simulink model "passive_filters"  (R2016a)
settings: Solver=ode23t  StartTime=0.0  StopTime=0.1  RelTol=1e-3  AbsTol=1e-3
libraries: fl_lib x60, nesl_utility x39
settings Model: Creator=marin  LastModifiedBy=marin
settings DataIOCC: LimitDataPoints=on
settings DebuggingCC: AllowSymbolicDim=off
settings ConfigComp: CovModelRefEnable=Off  CovSFcnEnable=off
settings SimscapeCC: SimscapeLogType=all  SimscapeLogDataHistory=10000

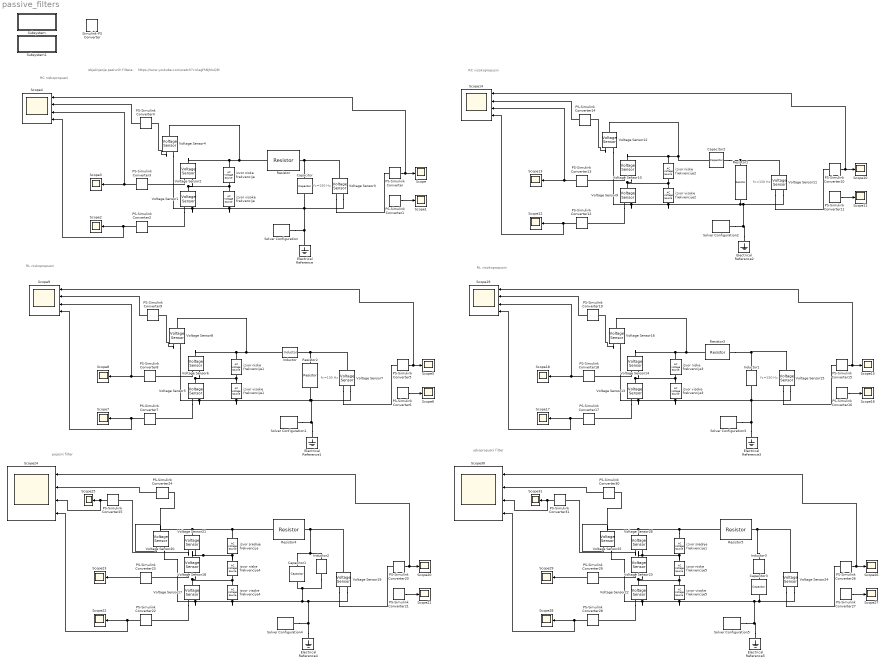
== system passive_filters ==
  note: uskopropusni filter
  note: pojasni filter
  note: RC visokopropusni
  note: RL niskopropusni
  note: RC niskopropusni
  note: objašnjenje pasivnih filtera:
  note: https://www.youtube.com/watch?v=lagfhNjMuQM
  note: fc=150 Hz
  note: fc=150 Hz
  note: fc=150 Hz
  note: RL visokopropusni
  note: fc=150 Hz
  Capacitor : fl_lib/Electrical/Electrical Elements/Capacitor  c=0.0011 F  r=1e-6 Ohm  g=0 1/Ohm  i_specify=off  i_priority=None  i=0 A  v_specify=off  v_priority=None  v=0 V  vc_specify=off  vc_priority=High  vc=0 V
  Capacitor1 : fl_lib/Electrical/Electrical Elements/Capacitor  c=0.0032 F  r=1e-6 Ohm  g=0 1/Ohm  i_specify=off  i_priority=None  i=0 A  v_specify=off  v_priority=None  v=0 V  vc_specify=off  vc_priority=High  vc=0 V
  Capacitor2 : fl_lib/Electrical/Electrical Elements/Capacitor  c=0.0011 F  r=1e-6 Ohm  g=0 1/Ohm  i_specify=off  i_priority=None  i=0 A  v_specify=off  v_priority=None  v=0 V  vc_specify=off  vc_priority=High  vc=0 V
  Capacitor3 : fl_lib/Electrical/Electrical Elements/Capacitor  c=0.0032 F  r=1e-6 Ohm  g=0 1/Ohm  i_specify=off  i_priority=None  i=0 A  v_specify=off  v_priority=None  v=0 V  vc_specify=off  vc_priority=High  vc=0 V
  Electrical Reference{,1..5} (6 alike) : fl_lib/Electrical/Electrical Elements/Electrical Reference
  Inductor : fl_lib/Electrical/Electrical Elements/Inductor  l=1e-6 H  r=0 Ohm  g=1e-9 1/Ohm  i_specify=off  i_priority=None  i=0 A  v_specify=off  v_priority=None  v=0 V  i_L_specify=off  i_L_priority=High  i_L=0 A
  Inductor1 : fl_lib/Electrical/Electrical Elements/Inductor  l=1e-6 H  r=0 Ohm  g=1e-9 1/Ohm  i_specify=off  i_priority=None  i=0 A  v_specify=off  v_priority=None  v=0 V  i_L_specify=off  i_L_priority=High  i_L=0 A
  Inductor2 : fl_lib/Electrical/Electrical Elements/Inductor  l=1.9894e-04 H  r=0 Ohm  g=1e-9 1/Ohm  i_specify=off  i_priority=None  i=0 A  v_specify=off  v_priority=None  v=0 V  i_L_specify=off  i_L_priority=High  i_L=0 A
  Inductor3 : fl_lib/Electrical/Electrical Elements/Inductor  l=1.9894e-04 H  r=0 Ohm  g=1e-9 1/Ohm  i_specify=off  i_priority=None  i=0 A  v_specify=off  v_priority=None  v=0 V  i_L_specify=off  i_L_priority=High  i_L=0 A
  PS-Simulink Converter{,1..31} (32 alike) : nesl_utility/PS-Simulink Converter  PhysicalDomain=network_engine_domain  SubClassName=ps_output  LeftPortType=input  RightPortType=output  PseudoPeriodic=off  Frequencies=[]  Unit=1  AffineConversion=off
  Resistor{,1,4..5} (4 alike) : fl_lib/Electrical/Electrical Elements/Resistor  R=1 Ohm  i_specify=off  i_priority=None  i=0 A  v_specify=off  v_priority=None  v=0 V
  Resistor2 : fl_lib/Electrical/Electrical Elements/Resistor  R=0.0011 Ohm  i_specify=off  i_priority=None  i=0 A  v_specify=off  v_priority=None  v=0 V
  Resistor3 : fl_lib/Electrical/Electrical Elements/Resistor  R=0.0011 Ohm  i_specify=off  i_priority=None  i=0 A  v_specify=off  v_priority=None  v=0 V
  Scope{,1..3,5..8,10..13,15..18,20..23,25..29,31} (26 alike) : Scope
  Scope{4,9,14,19,24,30} (6 alike) : Scope  NumInputPorts=4
  Simulink-PS Converter : nesl_utility/Simulink-PS Converter  PhysicalDomain=network_engine_domain  SubClassName=ps_input  LeftPortType=input  RightPortType=output  PseudoPeriodic=off  Frequencies=[]  NoiseDistribution=none  NoiseParameters=[]  Unit=1  AffineConversion=off  InputFiltering=off  SimscapeFilterOrder=1  InputFilterTimeConstant=0.001  UdotUserProvided=1
  Solver Configuration{,1..5} (6 alike) : nesl_utility/Solver Configuration  PhysicalDomain=network_engine_domain  SubClassName=solver  LeftPortType=input  RightPortType=generic  Accelerate=off  Tones=[]  Harmonics=[]  SimulateNoise=off  Profile=off  UseLocalSampling=off  EnableSwitchedLinearOptims=on  FrequencyDomain=off  UseCCode=off  RelTol=0.001  AbsTol=1e-06  MinStep=1e-09  ToWorkspace=off  RevertToSquareIcSolve=off  NumHomotopyIterations=100  PhasorMode=off  PhasorModeNumHarmonics=1  OverrideAbsTol=off  DoDC=off  ResidualTolerance=1e-09  UseLocalSolver=off  LocalSolverChoice=NE_BACKWARD_EULER_ADVANCER  LocalSolverSampleTime=0.001  DoFixedCost=off  MaxNonlinIter=3  MaxModeIter=2  LinearAlgebra=Sparse  DelaysMemoryBudget=1024  AutomaticFiltering=on  FilteringTimeConstant=0.001
  Subsystem : Subsystem
      settings: OpenFcn=open_system('simscape')
      mask Display: disp(sprintf('Open Simscape\nLibrary'));
  Subsystem1 : Subsystem
      settings: OpenFcn=|
      | load_system('fl_lib');
      | open_system('fl_lib/Electrical');
      mask Display: disp(sprintf('Open Electrical\nLibrary'));
  Voltage Sensor{1..26} (26 alike) : fl_lib/Electrical/Electrical Sensors/Voltage Sensor
  izvor niske frekvencije{,1..5} (6 alike) : fl_lib/Electrical/Electrical Sources/AC Voltage Source  amp=5 V  shift=0 deg  frequency=10 Hz  omega=0 rad/s
  izvor srednje frekvencije : fl_lib/Electrical/Electrical Sources/AC Voltage Source  amp=5 V  shift=0 deg  frequency=500 Hz  omega=0 rad/s
  izvor srednje frekvencije1 : fl_lib/Electrical/Electrical Sources/AC Voltage Source  amp=15 V  shift=0 deg  frequency=500 Hz  omega=0 rad/s
  izvor visoke frekvencije{,1..5} (6 alike) : fl_lib/Electrical/Electrical Sources/AC Voltage Source  amp=5 V  shift=0 deg  frequency=900 Hz  omega=0 rad/s
  wires:
  PS-Simulink Converter/1 -> Scope4/1, Scope/1
  PS-Simulink Converter1/1 -> Scope1/1
  PS-Simulink Converter2/1 -> Scope4/4, Scope2/1
  PS-Simulink Converter3/1 -> Scope4/3, Scope3/1
  PS-Simulink Converter4/1 -> Scope4/2
  PS-Simulink Converter5/1 -> Scope9/1, Scope5/1
  PS-Simulink Converter6/1 -> Scope6/1
  PS-Simulink Converter7/1 -> Scope9/4, Scope7/1
  PS-Simulink Converter8/1 -> Scope9/3, Scope8/1
  PS-Simulink Converter9/1 -> Scope9/2
  PS-Simulink Converter10/1 -> Scope14/1, Scope10/1
  PS-Simulink Converter11/1 -> Scope11/1
  PS-Simulink Converter12/1 -> Scope14/4, Scope12/1
  PS-Simulink Converter13/1 -> Scope14/3, Scope13/1
  PS-Simulink Converter14/1 -> Scope14/2
  PS-Simulink Converter15/1 -> Scope19/1, Scope15/1
  PS-Simulink Converter16/1 -> Scope16/1
  PS-Simulink Converter17/1 -> Scope19/4, Scope17/1
  PS-Simulink Converter18/1 -> Scope19/3, Scope18/1
  PS-Simulink Converter19/1 -> Scope19/2
  PS-Simulink Converter20/1 -> Scope24/1, Scope20/1
  PS-Simulink Converter21/1 -> Scope21/1
  PS-Simulink Converter22/1 -> Scope24/4, Scope22/1
  PS-Simulink Converter23/1 -> Scope23/1
  PS-Simulink Converter24/1 -> Scope24/2
  PS-Simulink Converter25/1 -> Scope24/3, Scope25/1
  PS-Simulink Converter26/1 -> Scope30/1, Scope26/1
  PS-Simulink Converter27/1 -> Scope27/1
  PS-Simulink Converter28/1 -> Scope30/4, Scope28/1
  PS-Simulink Converter29/1 -> Scope29/1
  PS-Simulink Converter30/1 -> Scope30/2
  PS-Simulink Converter31/1 -> Scope30/3, Scope31/1
  connections:
  Capacitor/LConn1 -- Voltage Sensor3/LConn1 -- Resistor/RConn1
  izvor visoke frekvencije/LConn1 -- Voltage Sensor2/RConn2 -- Voltage Sensor1/LConn1 -- izvor niske frekvencije/RConn1
  izvor niske frekvencije/LConn1 -- Voltage Sensor2/LConn1 -- Voltage Sensor4/LConn1 -- Resistor/LConn1
  Solver Configuration/RConn1 -- Voltage Sensor4/RConn2 -- Voltage Sensor1/RConn2 -- izvor visoke frekvencije/RConn1 -- Capacitor/RConn1 -- Voltage Sensor3/RConn2 -- Electrical Reference/LConn1
  Voltage Sensor1/RConn1 -- PS-Simulink Converter2/LConn1
  Voltage Sensor2/RConn1 -- PS-Simulink Converter3/LConn1
  Voltage Sensor3/RConn1 -- PS-Simulink Converter/LConn1
  Voltage Sensor4/RConn1 -- PS-Simulink Converter4/LConn1
  Voltage Sensor7/LConn1 -- Inductor/RConn1 -- Resistor2/LConn1
  izvor niske frekvencije1/RConn1 -- izvor visoke frekvencije1/LConn1 -- Voltage Sensor6/RConn2 -- Voltage Sensor5/LConn1
  Voltage Sensor8/LConn1 -- Inductor/LConn1 -- izvor niske frekvencije1/LConn1 -- Voltage Sensor6/LConn1
  Electrical Reference1/LConn1 -- Solver Configuration1/RConn1 -- Voltage Sensor7/RConn2 -- Voltage Sensor8/RConn2 -- Voltage Sensor5/RConn2 -- izvor visoke frekvencije1/RConn1 -- Resistor2/RConn1
  Voltage Sensor7/RConn1 -- PS-Simulink Converter5/LConn1
  Voltage Sensor8/RConn1 -- PS-Simulink Converter9/LConn1
  Voltage Sensor6/RConn1 -- PS-Simulink Converter8/LConn1
  Voltage Sensor5/RConn1 -- PS-Simulink Converter7/LConn1
  Voltage Sensor11/LConn1 -- Capacitor2/LConn1 -- Resistor1/LConn1
  izvor niske frekvencije2/RConn1 -- izvor visoke frekvencije2/LConn1 -- Voltage Sensor10/RConn2 -- Voltage Sensor9/LConn1
  izvor niske frekvencije2/LConn1 -- Voltage Sensor10/LConn1 -- Voltage Sensor12/LConn1 -- Capacitor2/RConn1
  Electrical Reference2/LConn1 -- Solver Configuration2/RConn1 -- Voltage Sensor11/RConn2 -- Voltage Sensor12/RConn2 -- Voltage Sensor9/RConn2 -- izvor visoke frekvencije2/RConn1 -- Resistor1/RConn1
  Voltage Sensor9/RConn1 -- PS-Simulink Converter12/LConn1
  Voltage Sensor11/RConn1 -- PS-Simulink Converter10/LConn1
  Voltage Sensor12/RConn1 -- PS-Simulink Converter14/LConn1
  Voltage Sensor10/RConn1 -- PS-Simulink Converter13/LConn1
  izvor niske frekvencije3/RConn1 -- izvor visoke frekvencije3/LConn1 -- Voltage Sensor14/RConn2 -- Voltage Sensor13/LConn1
  Voltage Sensor14/LConn1 -- izvor niske frekvencije3/LConn1 -- Resistor3/RConn1 -- Voltage Sensor16/LConn1
  Electrical Reference3/LConn1 -- Solver Configuration3/RConn1 -- Voltage Sensor15/RConn2 -- Inductor1/RConn1 -- izvor visoke frekvencije3/RConn1 -- Voltage Sensor16/RConn2 -- Voltage Sensor13/RConn2
  Voltage Sensor15/RConn1 -- PS-Simulink Converter15/LConn1
  Voltage Sensor13/RConn1 -- PS-Simulink Converter17/LConn1
  Voltage Sensor14/RConn1 -- PS-Simulink Converter18/LConn1
  Voltage Sensor16/RConn1 -- PS-Simulink Converter19/LConn1
  Inductor1/LConn1 -- Resistor3/LConn1 -- Voltage Sensor15/LConn1
  Resistor4/RConn1 -- Capacitor1/LConn1 -- Inductor2/LConn1 -- Voltage Sensor19/LConn1
  izvor niske frekvencije4/RConn1 -- izvor visoke frekvencije4/LConn1 -- Voltage Sensor18/RConn2 -- Voltage Sensor17/LConn1
  Voltage Sensor18/LConn1 -- Voltage Sensor21/RConn2 -- izvor srednje frekvencije/RConn1 -- izvor niske frekvencije4/LConn1
  Electrical Reference4/LConn1 -- Solver Configuration4/RConn1 -- Voltage Sensor19/RConn2 -- Voltage Sensor20/RConn2 -- Voltage Sensor17/RConn2 -- izvor visoke frekvencije4/RConn1 -- Capacitor1/RConn1 -- Inductor2/RConn1
  Voltage Sensor20/RConn1 -- PS-Simulink Converter24/LConn1
  Voltage Sensor17/RConn1 -- PS-Simulink Converter22/LConn1
  Voltage Sensor19/RConn1 -- PS-Simulink Converter20/LConn1
  Voltage Sensor18/RConn1 -- PS-Simulink Converter23/LConn1
  Voltage Sensor21/LConn1 -- Resistor4/LConn1 -- izvor srednje frekvencije/LConn1 -- Voltage Sensor20/LConn1
  Voltage Sensor21/RConn1 -- PS-Simulink Converter25/LConn1
  Resistor5/RConn1 -- Inductor3/LConn1 -- Voltage Sensor24/LConn1
  izvor niske frekvencije5/RConn1 -- izvor visoke frekvencije5/LConn1 -- Voltage Sensor23/RConn2 -- Voltage Sensor22/LConn1
  izvor niske frekvencije5/LConn1 -- Voltage Sensor26/RConn2 -- Voltage Sensor23/LConn1 -- izvor srednje frekvencije1/RConn1
  Electrical Reference5/LConn1 -- Solver Configuration5/RConn1 -- Capacitor3/RConn1 -- Voltage Sensor24/RConn2 -- izvor visoke frekvencije5/RConn1 -- Voltage Sensor25/RConn2 -- Voltage Sensor22/RConn2
  izvor srednje frekvencije1/LConn1 -- Voltage Sensor25/LConn1 -- Voltage Sensor26/LConn1 -- Resistor5/LConn1
  Voltage Sensor23/RConn1 -- PS-Simulink Converter29/LConn1
  Voltage Sensor24/RConn1 -- PS-Simulink Converter26/LConn1
  Voltage Sensor26/RConn1 -- PS-Simulink Converter31/LConn1
  Voltage Sensor25/RConn1 -- PS-Simulink Converter30/LConn1
  Voltage Sensor22/RConn1 -- PS-Simulink Converter28/LConn1
  Capacitor3/LConn1 -- Inductor3/RConn1

== system passive_filters/Subsystem ==

== system passive_filters/Subsystem1 ==
